simulink model "myModel"  (R2023b)
settings: Solver=VariableStepAuto  StartTime=0.0  StopTime=10  RelTol=1e-3
values from neighbouring files (symbols this model uses):
  A = [0, 0               ,   1           , 0 ... (first row only)    [mytask.m]
  B = [0, 0,  1/mc,   1/(L*mc)]'    [mytask.m]
  C = [1, 0,  0,  0]    [mytask.m]
  x0 = [0;    5*pi/180;   0;  0]    [mytask.m]
settings Model: Creator=admin  LastModifiedBy=admin

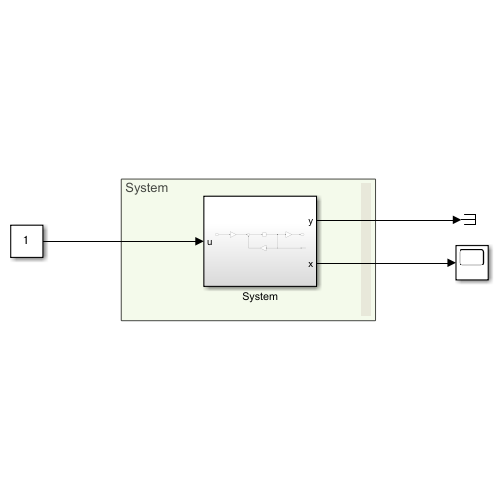
[thumbnail: Simulink's stored preview of the top-level diagram]
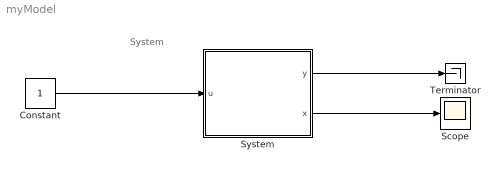
== system myModel ==
  note: System
  Constant : Constant
  Scope : Scope
  System : Subsystem
  Terminator : Terminator
  wires:
  System/1(y) -> Terminator/1
  System/2(x) -> Scope/1
  Constant/1 -> System/1(u)

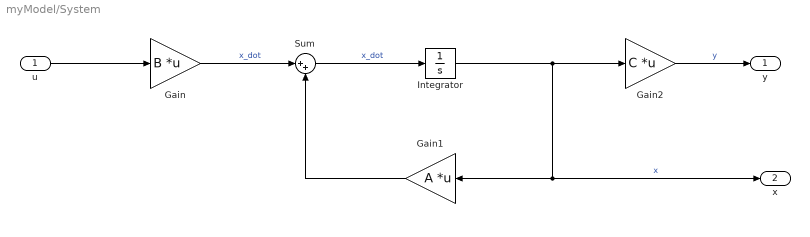
== system myModel/System ==
  u : Inport
  Gain : Gain  Gain=B  Multiplication=Matrix(K*u)
  Gain1 : Gain  Gain=A  Multiplication=Matrix(K*u)
  Gain2 : Gain  Gain=C  Multiplication=Matrix(K*u)
  Integrator : Integrator  InitialCondition=x0
  Sum : Sum  Inputs=|++
  y : Outport
  x : Outport  Port=2
  wires:
  Gain/1 -> Sum/1  "x_dot"
  Gain2/1 -> y/1  "y"
  Sum/1 -> Integrator/1  "x_dot"
  Gain1/1 -> Sum/2
  Integrator/1 -> x/1, Gain1/1, Gain2/1  "x"
  u/1 -> Gain/1
